simulink model "Change_Detection_Operators"  (R2024a)
settings: Solver=FixedStepDiscrete  StartTime=0.0  StopTime=10.0  FixedStep=1  RelTol=1e-3
libraries: simulink x1
settings Model: Creator=VICTUS  LastModifiedBy=VICTUS

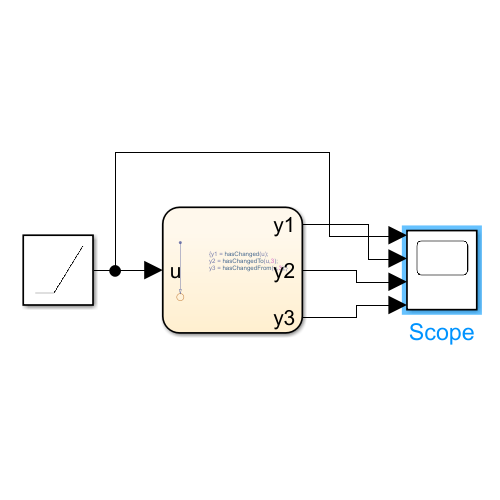
[thumbnail: Simulink's stored preview of the top-level diagram]
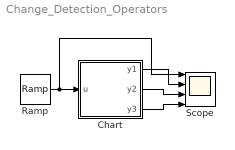
== system Change_Detection_Operators ==
  Chart : Stateflow chart  TreatAsAtomicUnit=on
  Ramp : simulink/Sources/Ramp  slope=1  start=0  InitialOutput=0
  Scope : Scope  NumInputPorts=4
  wires:
  Ramp/1 -> Scope/1, Chart/1(u)
  Chart/1(y1) -> Scope/2
  Chart/2(y2) -> Scope/3
  Chart/3(y3) -> Scope/4

== stateflow chart Change_Detection_Operators/Chart ==
  (default) -> (junction 14) : {y1 = hasChanged(u);
      | y2 = hasChangedTo(u,3);
      | y3 = hasChangedFrom(u,3);}
  data: y1 output double; y2 output double; y3 output double; u input double
